simulink model "UPS_3level_Ttype_Inverter_simplified_ctrl"  (R2012b)
settings: Solver=ode4  StartTime=0.0  StopTime=Tfinal  FixedStep=Ts  MaxStep=1e-5  RelTol=1e-3
values from neighbouring files (symbols this model uses):
  Ts = 1/(1*1e6)    (= 1e-06)    [Run.m]
  Vd = 720    [Run.m]
  VSI = rmfield(VSI, {'IF1', 'IF2', 'FLUXlin1', 'FLUXlin2',      'FLUXnonlin1', 'FLUXnonlin2', 'Lfnonlin'})    [Run.m]
undefined symbols (not defined in the file or in its folder): ADC, CTRL, DiscIntNeverNeededParam, PR, S, UPS
libraries: powerlib x113, simulink_extras x11, powerlib_extras x11, simulink x3
(part 1 of 3)
CloseFcn:
  | rtwprivate ssgencode ModelCloseRequest AC_DC_3f_400k_PW
settings Model: BufferReuse=off  Creator=Adam  LastModifiedBy=chstalm
settings DataIOCC: SignalLoggingSaveFormat=ModelDataLogs  InspectSignalLogs=on
settings OptimizationCC: BlockReduction=off  InlineParams=on  BufferReuse=off  InitFltsAndDblsToZero=on
settings DebuggingCC: SaveWithParameterizedLinksMsg=none  CheckSSInitialOutputMsg=off  SignalResolutionControl=TryResolveAllWithWarning  FcnCallInpInsideContextMsg=UseLocalSettings  UnconnectedInputMsg=none  UnconnectedOutputMsg=none  UnconnectedLineMsg=none  StrictBusMsg=Warning
settings GRTTargetCC: TargetFcnLib=ansi_tfl_tmw.mat  CombineOutputUpdateFcns=off  GRTInterface=on

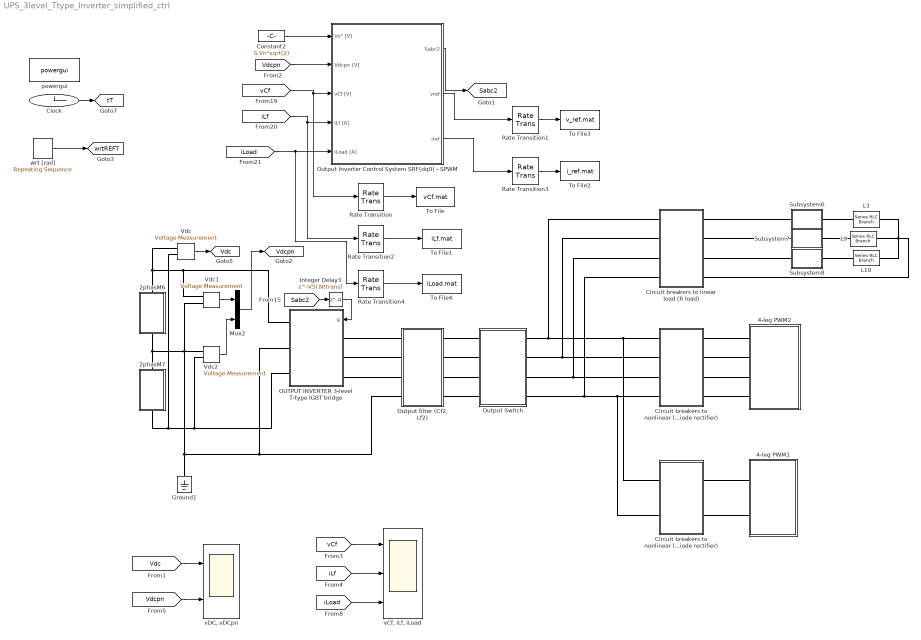
== system UPS_3level_Ttype_Inverter_simplified_ctrl ==
  2phasM6 : Subsystem
  2phasM7 : Subsystem
  4-leg PWM1 : Subsystem
  4-leg PWM2 : Subsystem
  Circuit breakers to linear load (R load) : Subsystem
  Circuit breakers to nonlinear load (1-phase diode rectifier) : Subsystem
  Circuit breakers to nonlinear load (3-phase diode rectifier) : Subsystem
  Clock : Clock
  Constant2 : Constant  Value=S.Vn*sqrt(2)  SampleTime=Ts
  Ground1 : powerlib/Elements/Ground  LConnTagsString=a
  Integer Delay3 : Delay  DelayLength=VSI.Nttransf  InitialCondition=0  InputProcessing=Inherited
  L10 : powerlib/Elements/Series RLC Branch  LConnTagsString=__new0  RConnTagsString=__new0  BranchType=RL  Resistance=VSI.Rc  Inductance=VSI.Lc  SetiL0=off  InitialCurrent=0  Capacitance=1.0  Setx0=off  InitialVoltage=0  Measurements=None
  L3 : powerlib/Elements/Series RLC Branch  LConnTagsString=__new0  RConnTagsString=__new0  BranchType=RL  Resistance=VSI.Ra  Inductance=VSI.La  SetiL0=off  InitialCurrent=0  Capacitance=1.0  Setx0=off  InitialVoltage=0  Measurements=None
  L9 : powerlib/Elements/Series RLC Branch  LConnTagsString=__new0  RConnTagsString=__new0  BranchType=RL  Resistance=VSI.Rb  Inductance=VSI.Lb  SetiL0=off  InitialCurrent=0  Capacitance=1.0  Setx0=off  InitialVoltage=0  Measurements=None
  Mux2 : Mux  Inputs=2
  OUTPUT INVERTER 3-level T-type IGBT bridge : Subsystem
  Output Switch : Subsystem
  "Output Inverter Control System SRF(dq0) - SPWM " : Subsystem
  "Output filter (Cf2, Lf2)" : Subsystem
  Rate Transition{,1..4} (5 alike) : RateTransition  OutPortSampleTime=1e-5
  Subsystem6 : Subsystem
  Subsystem7 : Subsystem
  Subsystem8 : Subsystem
  To File : ToFile  Filename=vCf.mat  MatrixName=vCf  SaveFormat=Timeseries
  To File1 : ToFile  Filename=iLf.mat  MatrixName=iLf  SaveFormat=Timeseries
  To File2 : ToFile  Filename=i_ref.mat  MatrixName=i_ref  SaveFormat=Timeseries
  To File3 : ToFile  Filename=v_ref.mat  MatrixName=v_ref  SaveFormat=Timeseries
  To File4 : ToFile  Filename=iLoad.mat  MatrixName=iLoad  SaveFormat=Timeseries
  Vdc : powerlib/Measurements/Voltage Measurement  PhasorSimulation=off  OutputType=Complex  PSBequivalent=0
  Vdc1 : powerlib/Measurements/Voltage Measurement  PhasorSimulation=off  OutputType=Complex  PSBequivalent=0
  Vdc2 : powerlib/Measurements/Voltage Measurement  PhasorSimulation=off  OutputType=Complex  PSBequivalent=0
  powergui : powerlib/powergui  SimulationMode=Discrete  SolverType=Tustin  SampleTime=Ts  frequency=60  SPID=off  DisableSnubberDevices=off  DisableRonSwitches=off  DisableVfSwitches=off  SwTol=0  Interpol=off  DisplayEquations=off  FunctionMessages=off  frequencyindice=0  Pbase=100e6  ErrMax=1e-4  Iterations=50  UnitsV=kV  UnitsW=MW  echomessages=off  HookPort=off  EnableUseOfTLC=off  x0status=blocks  RestoreLinks=warning  ResistiveCurrentMeasurement=off  Frange=[0:2:500]  Ylog=off  Xlog=on  ShowGrid=off  save=off  variable=ZData  ZoomFFT=on  StartTime=0.0  cycles=1  DisplayStyle=1  fundamental=60  FreqAxis=off  MaxFrequency=1000  frequencyindicesteady=1  RmsSteady=1  display=off  Ts=0  methode=off
  "vCf, iLf, iLoad" : Scope  NumInputPorts=3
      settings: TimeRange=0.7000000000000001  YMin=-500~-400~-400  YMax=500~400~400  SaveName=VSIout  DataFormat=Structure  Decimation=10  SampleInput=on
  "vDC, vDCpn" : Scope  NumInputPorts=2
      settings: TimeRange=0.1738072054527751  YMin=0~0  YMax=750~375  SaveName=Rectifier_in1  DataFormat=Structure  Decimation=10  SampleInput=on
  wrt [rad] : simulink/Sources/Repeating Sequence  rep_seq_t="[0    1/S.fn]"  rep_seq_y="[0    2*pi]"
  tag scope: Sabc2=global, Vdc=global, Vdcpn=global, tT=global, wrtREFT=global
  wires:
  Clock/1 -> [tT]
  [Sabc2] -> Integer Delay3/1
  [Vdcpn] -> "Output Inverter Control System SRF(dq0) - SPWM "/2(Vdcpn [V])
  [vCf] -> Rate Transition/1, "Output Inverter Control System SRF(dq0) - SPWM "/3(vCf [V])
  [iLf] -> Rate Transition2/1, "Output Inverter Control System SRF(dq0) - SPWM "/4(iLf [A])
  "Output Inverter Control System SRF(dq0) - SPWM "/1(Sabc2) -> [Sabc2]
  [iLoad] -> Rate Transition4/1, "Output Inverter Control System SRF(dq0) - SPWM "/5(iLoad [A])
  Integer Delay3/1 -> OUTPUT INVERTER 3-level T-type IGBT bridge/1(g)
  Vdc/1 -> [Vdc]
  [vCf] -> "vCf, iLf, iLoad"/1
  [iLoad] -> "vCf, iLf, iLoad"/3
  [iLf] -> "vCf, iLf, iLoad"/2
  Vdc1/1 -> Mux2/1
  Vdc2/1 -> Mux2/2
  Mux2/1 -> [Vdcpn]
  [Vdcpn] -> "vDC, vDCpn"/2
  [Vdc] -> "vDC, vDCpn"/1
  wrt [rad]/1 -> [wrtREFT]
  Rate Transition/1 -> To File/1
  Rate Transition1/1 -> To File3/1
  "Output Inverter Control System SRF(dq0) - SPWM "/2(vref) -> Rate Transition1/1
  Constant2/1 -> "Output Inverter Control System SRF(dq0) - SPWM "/1(Vs* [V])
  Rate Transition2/1 -> To File1/1
  Rate Transition3/1 -> To File2/1
  "Output Inverter Control System SRF(dq0) - SPWM "/3(iref) -> Rate Transition3/1
  Rate Transition4/1 -> To File4/1
  connections:
  Output Switch/LConn1 -- "Output filter (Cf2, Lf2)"/RConn1
  Output Switch/LConn2 -- "Output filter (Cf2, Lf2)"/RConn2
  Output Switch/LConn4 -- "Output filter (Cf2, Lf2)"/RConn4
  Output Switch/LConn3 -- "Output filter (Cf2, Lf2)"/RConn3
  Vdc2/LConn2 -- OUTPUT INVERTER 3-level T-type IGBT bridge/RConn3 -- 2phasM7/RConn1 -- Vdc/LConn2
  Vdc1/LConn1 -- OUTPUT INVERTER 3-level T-type IGBT bridge/RConn1 -- 2phasM6/LConn1 -- Vdc/LConn1
  OUTPUT INVERTER 3-level T-type IGBT bridge/LConn1 -- "Output filter (Cf2, Lf2)"/LConn1
  OUTPUT INVERTER 3-level T-type IGBT bridge/LConn2 -- "Output filter (Cf2, Lf2)"/LConn2
  OUTPUT INVERTER 3-level T-type IGBT bridge/LConn3 -- "Output filter (Cf2, Lf2)"/LConn3
  OUTPUT INVERTER 3-level T-type IGBT bridge/RConn2 -- "Output filter (Cf2, Lf2)"/LConn4 -- Ground1/LConn1 -- Vdc2/LConn1 -- Vdc1/LConn2 -- 2phasM7/LConn1 -- 2phasM6/RConn1
  Subsystem6/RConn1 -- L3/LConn1
  Subsystem8/RConn1 -- L10/LConn1
  Subsystem7/RConn1 -- L9/LConn1
  Circuit breakers to linear load (R load)/RConn1 -- Subsystem6/LConn1
  Circuit breakers to linear load (R load)/RConn2 -- Subsystem7/LConn1
  Circuit breakers to linear load (R load)/RConn3 -- Subsystem8/LConn1
  L10/RConn1 -- L3/RConn1 -- L9/RConn1 -- Circuit breakers to linear load (R load)/RConn4
  Circuit breakers to nonlinear load (3-phase diode rectifier)/RConn1 -- 4-leg PWM2/LConn1
  Circuit breakers to nonlinear load (3-phase diode rectifier)/RConn2 -- 4-leg PWM2/LConn2
  Circuit breakers to nonlinear load (3-phase diode rectifier)/RConn3 -- 4-leg PWM2/LConn3
  Circuit breakers to nonlinear load (3-phase diode rectifier)/RConn4 -- 4-leg PWM2/LConn4
  4-leg PWM1/LConn1 -- Circuit breakers to nonlinear load (1-phase diode rectifier)/RConn1
  4-leg PWM1/LConn2 -- Circuit breakers to nonlinear load (1-phase diode rectifier)/RConn2
  Output Switch/RConn1 -- Circuit breakers to nonlinear load (1-phase diode rectifier)/LConn1 -- Circuit breakers to nonlinear load (3-phase diode rectifier)/LConn1 -- Circuit breakers to linear load (R load)/LConn1
  Output Switch/RConn2 -- Circuit breakers to nonlinear load (3-phase diode rectifier)/LConn2 -- Circuit breakers to linear load (R load)/LConn2
  Output Switch/RConn3 -- Circuit breakers to nonlinear load (3-phase diode rectifier)/LConn3 -- Circuit breakers to linear load (R load)/LConn3
  Output Switch/RConn4 -- Circuit breakers to nonlinear load (1-phase diode rectifier)/LConn2 -- Circuit breakers to nonlinear load (3-phase diode rectifier)/LConn4 -- Circuit breakers to linear load (R load)/LConn4

== system UPS_3level_Ttype_Inverter_simplified_ctrl/2phasM6 ==
  DC Voltage Source : powerlib/Electrical Sources/DC Voltage Source  Amplitude=Vd/2  Measurements=None
  Vd1 : powerlib/Measurements/Voltage Measurement  PhasorSimulation=off  OutputType=Complex  PSBequivalent=0
  DC+ : PMIOPort  Port=1  Side=Left
  n : PMIOPort  Port=2  Side=Right
  tag scope: Vd1T=global
  wires:
  Vd1/1 -> [Vd1T]
  connections:
  DC+/RConn1 -- DC Voltage Source/RConn1 -- Vd1/LConn1
  n/RConn1 -- DC Voltage Source/LConn1 -- Vd1/LConn2

== system UPS_3level_Ttype_Inverter_simplified_ctrl/2phasM7 ==
  DC Voltage Source : powerlib/Electrical Sources/DC Voltage Source  Amplitude=Vd/2  Measurements=None
  Vd2 : powerlib/Measurements/Voltage Measurement  PhasorSimulation=off  OutputType=Complex  PSBequivalent=0
  n : PMIOPort  Port=1  Side=Left
  DC- : PMIOPort  Port=2  Side=Right
  tag scope: Vd2T=global
  wires:
  Vd2/1 -> [Vd2T]
  connections:
  n/RConn1 -- DC Voltage Source/RConn1 -- Vd2/LConn1
  DC-/RConn1 -- DC Voltage Source/LConn1 -- Vd2/LConn2

== system UPS_3level_Ttype_Inverter_simplified_ctrl/4-leg PWM1 ==
  D{1..2,7..8} (4 alike) : powerlib/Power Electronics/Diode  Ron=1e-3  Lon=0  Vf=0.8  IC=0  UseSnubber=off  Rs=1e6  Cs=inf  Measurements=off
  L1 : powerlib/Elements/Series RLC Branch  LConnTagsString=__new0  RConnTagsString=__new0  BranchType=R  Resistance=VSI.DR_Rs  Inductance=VSI.La  SetiL0=off  InitialCurrent=0  Capacitance=1.0  Setx0=off  InitialVoltage=0  Measurements=None
  L7 : powerlib/Elements/Series RLC Branch  LConnTagsString=__new0  RConnTagsString=__new0  BranchType=R  Resistance=VSI.DR_Rload  Inductance=VSI.La  SetiL0=off  InitialCurrent=0  Capacitance=1.0  Setx0=off  InitialVoltage=0  Measurements=None
  Series RLC Branch1 : powerlib/Elements/Series RLC Branch  LConnTagsString=__new0  RConnTagsString=__new0  BranchType=C  Resistance=1  Inductance=1e-3  SetiL0=off  InitialCurrent=0  Capacitance=VSI.DR_C  Setx0=on  InitialVoltage=VSI.DR_Vc0  Measurements=None
  Subsystem3 : Subsystem
  A : PMIOPort  Tag=PMCPort  Port=1  Side=Left
  N : PMIOPort  Tag=PMCPort  Port=2  Side=Left
  connections:
  D1/RConn1 -- Series RLC Branch1/LConn1 -- L7/LConn1 -- D7/RConn1
  D2/RConn1 -- L1/LConn1 -- D1/LConn1
  D8/LConn1 -- Series RLC Branch1/RConn1 -- L7/RConn1 -- D2/LConn1
  Subsystem3/LConn1 -- A/RConn1
  Subsystem3/RConn1 -- L1/RConn1
  D8/RConn1 -- N/RConn1 -- D7/LConn1

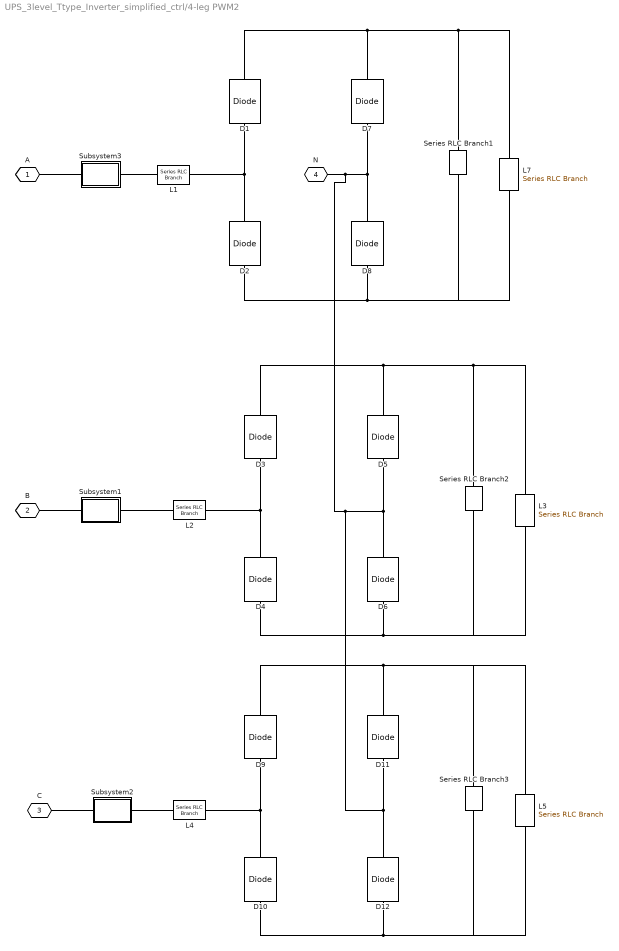
== system UPS_3level_Ttype_Inverter_simplified_ctrl/4-leg PWM2 ==
  D{1..12} (12 alike) : powerlib/Power Electronics/Diode  Ron=1e-3  Lon=0  Vf=0.8  IC=0  UseSnubber=off  Rs=1e6  Cs=inf  Measurements=off
  L1 : powerlib/Elements/Series RLC Branch  LConnTagsString=__new0  RConnTagsString=__new0  BranchType=R  Resistance=VSI.DR_Rs  Inductance=VSI.La  SetiL0=off  InitialCurrent=0  Capacitance=1.0  Setx0=off  InitialVoltage=0  Measurements=None
  L2 : powerlib/Elements/Series RLC Branch  LConnTagsString=__new0  RConnTagsString=__new0  BranchType=R  Resistance=VSI.DR_Rs  Inductance=VSI.La  SetiL0=off  InitialCurrent=0  Capacitance=1.0  Setx0=off  InitialVoltage=0  Measurements=None
  L3 : powerlib/Elements/Series RLC Branch  LConnTagsString=__new0  RConnTagsString=__new0  BranchType=R  Resistance=VSI.DR_Rload  Inductance=VSI.La  SetiL0=off  InitialCurrent=0  Capacitance=1.0  Setx0=off  InitialVoltage=0  Measurements=None
  L4 : powerlib/Elements/Series RLC Branch  LConnTagsString=__new0  RConnTagsString=__new0  BranchType=R  Resistance=VSI.DR_Rs  Inductance=VSI.La  SetiL0=off  InitialCurrent=0  Capacitance=1.0  Setx0=off  InitialVoltage=0  Measurements=None
  L5 : powerlib/Elements/Series RLC Branch  LConnTagsString=__new0  RConnTagsString=__new0  BranchType=R  Resistance=VSI.DR_Rload  Inductance=VSI.La  SetiL0=off  InitialCurrent=0  Capacitance=1.0  Setx0=off  InitialVoltage=0  Measurements=None
  L7 : powerlib/Elements/Series RLC Branch  LConnTagsString=__new0  RConnTagsString=__new0  BranchType=R  Resistance=VSI.DR_Rload  Inductance=VSI.La  SetiL0=off  InitialCurrent=0  Capacitance=1.0  Setx0=off  InitialVoltage=0  Measurements=None
  Series RLC Branch1 : powerlib/Elements/Series RLC Branch  LConnTagsString=__new0  RConnTagsString=__new0  BranchType=C  Resistance=1  Inductance=1e-3  SetiL0=off  InitialCurrent=0  Capacitance=VSI.DR_C  Setx0=on  InitialVoltage=VSI.DR_Vc0  Measurements=None
  Series RLC Branch2 : powerlib/Elements/Series RLC Branch  LConnTagsString=__new0  RConnTagsString=__new0  BranchType=C  Resistance=1  Inductance=1e-3  SetiL0=off  InitialCurrent=0  Capacitance=VSI.DR_C  Setx0=on  InitialVoltage=VSI.DR_Vc0  Measurements=None
  Series RLC Branch3 : powerlib/Elements/Series RLC Branch  LConnTagsString=__new0  RConnTagsString=__new0  BranchType=C  Resistance=1  Inductance=1e-3  SetiL0=off  InitialCurrent=0  Capacitance=VSI.DR_C  Setx0=on  InitialVoltage=VSI.DR_Vc0  Measurements=None
  Subsystem1 : Subsystem
  Subsystem2 : Subsystem
  Subsystem3 : Subsystem
  A : PMIOPort  Tag=PMCPort  Port=1  Side=Left
  B : PMIOPort  Tag=PMCPort  Port=2  Side=Left
  C : PMIOPort  Tag=PMCPort  Port=3  Side=Left
  N : PMIOPort  Tag=PMCPort  Port=4  Side=Left
  connections:
  D1/RConn1 -- L7/LConn1 -- Series RLC Branch1/LConn1 -- D7/RConn1
  D2/RConn1 -- L1/LConn1 -- D1/LConn1
  D8/LConn1 -- L7/RConn1 -- Series RLC Branch1/RConn1 -- D2/LConn1
  D4/RConn1 -- L2/LConn1 -- D3/LConn1
  D6/LConn1 -- L3/RConn1 -- Series RLC Branch2/RConn1 -- D4/LConn1
  D9/RConn1 -- Series RLC Branch3/LConn1 -- L5/LConn1 -- D11/RConn1
  D10/RConn1 -- L4/LConn1 -- D9/LConn1
  D12/LConn1 -- L5/RConn1 -- Series RLC Branch3/RConn1 -- D10/LConn1
  D3/RConn1 -- L3/LConn1 -- Series RLC Branch2/LConn1 -- D5/RConn1
  Subsystem2/LConn1 -- C/RConn1
  Subsystem1/LConn1 -- B/RConn1
  Subsystem3/LConn1 -- A/RConn1
  Subsystem3/RConn1 -- L1/RConn1
  D12/RConn1 -- D11/LConn1 -- D6/RConn1 -- D5/LConn1 -- D8/RConn1 -- D7/LConn1 -- N/RConn1
  L2/RConn1 -- Subsystem1/RConn1
  L4/RConn1 -- Subsystem2/RConn1

== system UPS_3level_Ttype_Inverter_simplified_ctrl/Circuit breakers to linear load (R load) ==
  Branch_C : MultiPortSwitch  Inputs=4  SaturateOnIntegerOverflow=on  InputSameDT=on
  Constant1 : Constant  Value=[1 0 0 1]
  Constant2 : Constant  Value=UPS.LoadR123 + 1
  Constant3 : Constant  Value=[1 1 0 1]
  Constant4 : Constant  Value=[1 1 1 1]
  Constant5 : Constant  Value=[0 0 0 0]
  Data Type Conversion{1..4} (4 alike) : DataTypeConversion  OutDataTypeStr=boolean  SaturateOnIntegerOverflow=on  RndMeth=Zero
  Demux : Demux
  Ideal Switch{,1..3} (4 alike) : powerlib/Power Electronics/Ideal Switch  Ron=0.001  Lon=0  IC=0  Rs=1e6  Cs=inf  Measurements=off
  A2 : PMIOPort  Port=1  Side=Left
  B2 : PMIOPort  Port=2  Side=Left
  C2 : PMIOPort  Port=3  Side=Left
  N2 : PMIOPort  Port=4  Side=Left
  a2 : PMIOPort  Port=5  Side=Right
  b2 : PMIOPort  Port=6  Side=Right
  c2 : PMIOPort  Port=7  Side=Right
  n2 : PMIOPort  Port=8  Side=Right
  wires:
  Constant4/1 -> Branch_C/5
  Constant3/1 -> Branch_C/4
  Constant1/1 -> Branch_C/3
  Constant5/1 -> Branch_C/2
  Constant2/1 -> Branch_C/1
  Branch_C/1 -> Demux/1
  Data Type Conversion2/1 -> Ideal Switch3/1
  Data Type Conversion1/1 -> Ideal Switch2/1
  Data Type Conversion3/1 -> Ideal Switch1/1
  Data Type Conversion4/1 -> Ideal Switch/1
  Demux/1 -> Data Type Conversion2/1
  Demux/2 -> Data Type Conversion1/1
  Demux/3 -> Data Type Conversion3/1
  Demux/4 -> Data Type Conversion4/1
  connections:
  Ideal Switch/LConn1 -- N2/RConn1
  n2/RConn1 -- Ideal Switch/RConn1
  Ideal Switch1/LConn1 -- C2/RConn1
  Ideal Switch1/RConn1 -- c2/RConn1
  Ideal Switch2/LConn1 -- B2/RConn1
  Ideal Switch2/RConn1 -- b2/RConn1
  Ideal Switch3/LConn1 -- A2/RConn1
  Ideal Switch3/RConn1 -- a2/RConn1

== system UPS_3level_Ttype_Inverter_simplified_ctrl/Circuit breakers to nonlinear load (1-phase diode rectifier) ==
  Constant2 : Constant  Value=UPS.LoadD1
  Data Type Conversion2 : DataTypeConversion  OutDataTypeStr=boolean  SaturateOnIntegerOverflow=on  RndMeth=Zero
  Ideal Switch2 : powerlib/Power Electronics/Ideal Switch  Ron=0.001  Lon=0  IC=0  Rs=1e6  Cs=inf  Measurements=off
  Ideal Switch3 : powerlib/Power Electronics/Ideal Switch  Ron=0.001  Lon=0  IC=0  Rs=1e6  Cs=inf  Measurements=off
  A2 : PMIOPort  Port=1  Side=Left
  N2 : PMIOPort  Port=2  Side=Left
  a2 : PMIOPort  Port=3  Side=Right
  n2 : PMIOPort  Port=4  Side=Right
  wires:
  Constant2/1 -> Data Type Conversion2/1
  Data Type Conversion2/1 -> Ideal Switch3/1, Ideal Switch2/1
  connections:
  Ideal Switch2/LConn1 -- N2/RConn1
  Ideal Switch2/RConn1 -- n2/RConn1
  Ideal Switch3/LConn1 -- A2/RConn1
  Ideal Switch3/RConn1 -- a2/RConn1

== system UPS_3level_Ttype_Inverter_simplified_ctrl/Circuit breakers to nonlinear load (3-phase diode rectifier) ==
  Constant2 : Constant  Value=UPS.LoadD3
  Data Type Conversion2 : DataTypeConversion  OutDataTypeStr=boolean  SaturateOnIntegerOverflow=on  RndMeth=Zero
  Ideal Switch{,1..3} (4 alike) : powerlib/Power Electronics/Ideal Switch  Ron=0.001  Lon=0  IC=0  Rs=1e6  Cs=inf  Measurements=off
  A2 : PMIOPort  Port=1  Side=Left
  B2 : PMIOPort  Port=2  Side=Left
  C2 : PMIOPort  Port=3  Side=Left
  N2 : PMIOPort  Port=4  Side=Left
  a2 : PMIOPort  Port=5  Side=Right
  b2 : PMIOPort  Port=6  Side=Right
  c2 : PMIOPort  Port=7  Side=Right
  n2 : PMIOPort  Port=8  Side=Right
  wires:
  Constant2/1 -> Data Type Conversion2/1
  Data Type Conversion2/1 -> Ideal Switch3/1, Ideal Switch2/1, Ideal Switch1/1, Ideal Switch/1
  connections:
  Ideal Switch/LConn1 -- N2/RConn1
  n2/RConn1 -- Ideal Switch/RConn1
  Ideal Switch1/LConn1 -- C2/RConn1
  Ideal Switch1/RConn1 -- c2/RConn1
  Ideal Switch2/LConn1 -- B2/RConn1
  Ideal Switch2/RConn1 -- b2/RConn1
  Ideal Switch3/LConn1 -- A2/RConn1
  Ideal Switch3/RConn1 -- a2/RConn1

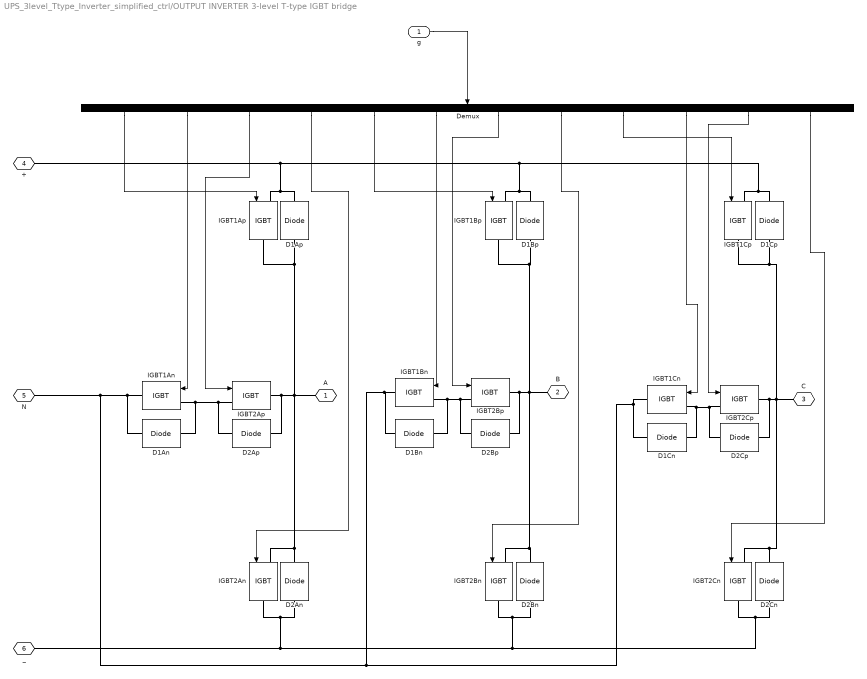
== system UPS_3level_Ttype_Inverter_simplified_ctrl/OUTPUT INVERTER 3-level T-type IGBT bridge ==
  g : Inport
  D1An : powerlib/Power Electronics/Diode  Ron=1e-3  Lon=0  Vf=0.8  IC=0  UseSnubber=off  Rs=inf  Cs=0  Measurements=off
  D1Ap : powerlib/Power Electronics/Diode  Ron=1e-3  Lon=0  Vf=0.8  IC=0  UseSnubber=off  Rs=inf  Cs=0  Measurements=off
  D1Bn : powerlib/Power Electronics/Diode  Ron=1e-3  Lon=0  Vf=0.8  IC=0  UseSnubber=off  Rs=inf  Cs=0  Measurements=off
  D1Bp : powerlib/Power Electronics/Diode  Ron=1e-3  Lon=0  Vf=0.8  IC=0  UseSnubber=off  Rs=inf  Cs=0  Measurements=off
  D1Cn : powerlib/Power Electronics/Diode  Ron=1e-3  Lon=0  Vf=0.8  IC=0  UseSnubber=off  Rs=inf  Cs=0  Measurements=off
  D1Cp : powerlib/Power Electronics/Diode  Ron=1e-3  Lon=0  Vf=0.8  IC=0  UseSnubber=off  Rs=inf  Cs=0  Measurements=off
  D2An : powerlib/Power Electronics/Diode  Ron=1e-3  Lon=0  Vf=0.8  IC=0  UseSnubber=off  Rs=inf  Cs=0  Measurements=off
  D2Ap : powerlib/Power Electronics/Diode  Ron=1e-3  Lon=0  Vf=0.8  IC=0  UseSnubber=off  Rs=inf  Cs=0  Measurements=off
  D2Bn : powerlib/Power Electronics/Diode  Ron=1e-3  Lon=0  Vf=0.8  IC=0  UseSnubber=off  Rs=inf  Cs=0  Measurements=off
  D2Bp : powerlib/Power Electronics/Diode  Ron=1e-3  Lon=0  Vf=0.8  IC=0  UseSnubber=off  Rs=inf  Cs=0  Measurements=off
  D2Cn : powerlib/Power Electronics/Diode  Ron=1e-3  Lon=0  Vf=0.8  IC=0  UseSnubber=off  Rs=inf  Cs=0  Measurements=off
  D2Cp : powerlib/Power Electronics/Diode  Ron=1e-3  Lon=0  Vf=0.8  IC=0  UseSnubber=off  Rs=inf  Cs=0  Measurements=off
  Demux : Demux  Outputs=12
  IGBT1An : powerlib/Power Electronics/IGBT  Ron=1e-3  Lon=0  Vf=1  Tf=0  Tt=0  IC=0  Rs=1e5  Cs=inf  Measurements=off
  IGBT1Ap : powerlib/Power Electronics/IGBT  Ron=1e-3  Lon=0  Vf=1  Tf=0  Tt=0  IC=0  Rs=1e5  Cs=inf  Measurements=off
  IGBT1Bn : powerlib/Power Electronics/IGBT  Ron=1e-3  Lon=0  Vf=1  Tf=0  Tt=0  IC=0  Rs=1e5  Cs=inf  Measurements=off
  IGBT1Bp : powerlib/Power Electronics/IGBT  Ron=1e-3  Lon=0  Vf=1  Tf=0  Tt=0  IC=0  Rs=1e5  Cs=inf  Measurements=off
  IGBT1Cn : powerlib/Power Electronics/IGBT  Ron=1e-3  Lon=0  Vf=1  Tf=0  Tt=0  IC=0  Rs=1e5  Cs=inf  Measurements=off
  IGBT1Cp : powerlib/Power Electronics/IGBT  Ron=1e-3  Lon=0  Vf=1  Tf=0  Tt=0  IC=0  Rs=1e5  Cs=inf  Measurements=off
  IGBT2An : powerlib/Power Electronics/IGBT  Ron=1e-3  Lon=0  Vf=1  Tf=0  Tt=0  IC=0  Rs=1e5  Cs=inf  Measurements=off
  IGBT2Ap : powerlib/Power Electronics/IGBT  Ron=1e-3  Lon=0  Vf=1  Tf=0  Tt=0  IC=0  Rs=1e5  Cs=inf  Measurements=off
  IGBT2Bn : powerlib/Power Electronics/IGBT  Ron=1e-3  Lon=0  Vf=1  Tf=0  Tt=0  IC=0  Rs=1e5  Cs=inf  Measurements=off
  IGBT2Bp : powerlib/Power Electronics/IGBT  Ron=1e-3  Lon=0  Vf=1  Tf=0  Tt=0  IC=0  Rs=1e5  Cs=inf  Measurements=off
  IGBT2Cn : powerlib/Power Electronics/IGBT  Ron=1e-3  Lon=0  Vf=1  Tf=0  Tt=0  IC=0  Rs=1e5  Cs=inf  Measurements=off
  IGBT2Cp : powerlib/Power Electronics/IGBT  Ron=1e-3  Lon=0  Vf=1  Tf=0  Tt=0  IC=0  Rs=1e5  Cs=inf  Measurements=off
  A : PMIOPort  Tag=PMCPort  Port=1  Side=Left
  B : PMIOPort  Tag=PMCPort  Port=2  Side=Left
  C : PMIOPort  Tag=PMCPort  Port=3  Side=Left
  + : PMIOPort  Tag=PMCPort  Port=4  Side=Right
  N : PMIOPort  Tag=PMCPort  Port=5  Side=Right
  _ : PMIOPort  Tag=PMCPort  Port=6  Side=Right
  wires:
  g/1 -> Demux/1
  Demux/1 -> IGBT1Ap/1
  Demux/2 -> IGBT1An/1
  Demux/3 -> IGBT2Ap/1
  Demux/4 -> IGBT2An/1
  Demux/5 -> IGBT1Bp/1
  Demux/6 -> IGBT1Bn/1
  Demux/7 -> IGBT2Bp/1
  Demux/8 -> IGBT2Bn/1
  Demux/9 -> IGBT1Cp/1
  Demux/10 -> IGBT1Cn/1
  Demux/11 -> IGBT2Cp/1
  Demux/12 -> IGBT2Cn/1
  connections:
  IGBT1Cp/LConn1 -- D1Cp/RConn1 -- IGBT1Ap/LConn1 -- D1Ap/RConn1 -- +/RConn1 -- D1Bp/RConn1 -- IGBT1Bp/LConn1
  IGBT2Ap/LConn1 -- D2Ap/RConn1 -- IGBT1An/LConn1 -- D1An/RConn1
  IGBT1Cp/RConn1 -- D1Cp/LConn1 -- D2Cp/LConn1 -- IGBT2Cp/RConn1 -- C/RConn1 -- IGBT2Cn/LConn1 -- D2Cn/RConn1
  IGBT2Cn/RConn1 -- D2Cn/LConn1 -- _/RConn1 -- IGBT2An/RConn1 -- D2An/LConn1 -- IGBT2Bn/RConn1 -- D2Bn/LConn1
  IGBT1Ap/RConn1 -- D1Ap/LConn1 -- IGBT2An/LConn1 -- D2An/RConn1 -- A/RConn1 -- IGBT2Ap/RConn1 -- D2Ap/LConn1
  D2Bp/RConn1 -- IGBT2Bp/LConn1 -- IGBT1Bn/LConn1 -- D1Bn/RConn1
  D2Bn/RConn1 -- IGBT2Bn/LConn1 -- D1Bp/LConn1 -- IGBT1Bp/RConn1 -- D2Bp/LConn1 -- IGBT2Bp/RConn1 -- B/RConn1
  D2Cp/RConn1 -- IGBT2Cp/LConn1 -- D1Cn/RConn1 -- IGBT1Cn/LConn1
  IGBT1Cn/RConn1 -- IGBT1An/RConn1 -- D1An/LConn1 -- N/RConn1 -- IGBT1Bn/RConn1 -- D1Bn/LConn1 -- D1Cn/LConn1

== system UPS_3level_Ttype_Inverter_simplified_ctrl/Output Switch ==
  2 [s]1 : Constant  Value=VSI.ton
  2 [s]5 : Constant  Value=VSI.tk
  Logical Operator : Logic  AllPortsSameDT=off  OutDataTypeStr=boolean
  Relational Operator1 : RelationalOperator  OutDataTypeStr=boolean
  Relational Operator3 : RelationalOperator  Operator=<=  OutDataTypeStr=boolean
  Subsystem4 : Subsystem
  Subsystem5 : Subsystem
  Subsystem7 : Subsystem
  A2 : PMIOPort  Port=1  Side=Left
  B2 : PMIOPort  Port=2  Side=Left
  a2 : PMIOPort  Port=3  Side=Right
  b2 : PMIOPort  Port=4  Side=Right
  C2 : PMIOPort  Port=5  Side=Left
  c2 : PMIOPort  Port=6  Side=Right
  N2 : PMIOPort  Port=7  Side=Left
  n2 : PMIOPort  Port=8  Side=Right
  wires:
  2 [s]1/1 -> Relational Operator1/2
  Relational Operator1/1 -> Logical Operator/1
  Relational Operator3/1 -> Logical Operator/2
  2 [s]5/1 -> Relational Operator3/2
  [tT] -> Relational Operator1/1, Relational Operator3/1
  Logical Operator/1 -> Subsystem5/1(on/off), Subsystem4/1(on/off), Subsystem7/1(on/off)
  connections:
  Subsystem4/RConn1 -- b2/RConn1
  N2/RConn1 -- n2/RConn1
  Subsystem7/RConn1 -- a2/RConn1
  Subsystem5/RConn1 -- c2/RConn1
  C2/RConn1 -- Subsystem5/LConn1
  B2/RConn1 -- Subsystem4/LConn1
  A2/RConn1 -- Subsystem7/LConn1

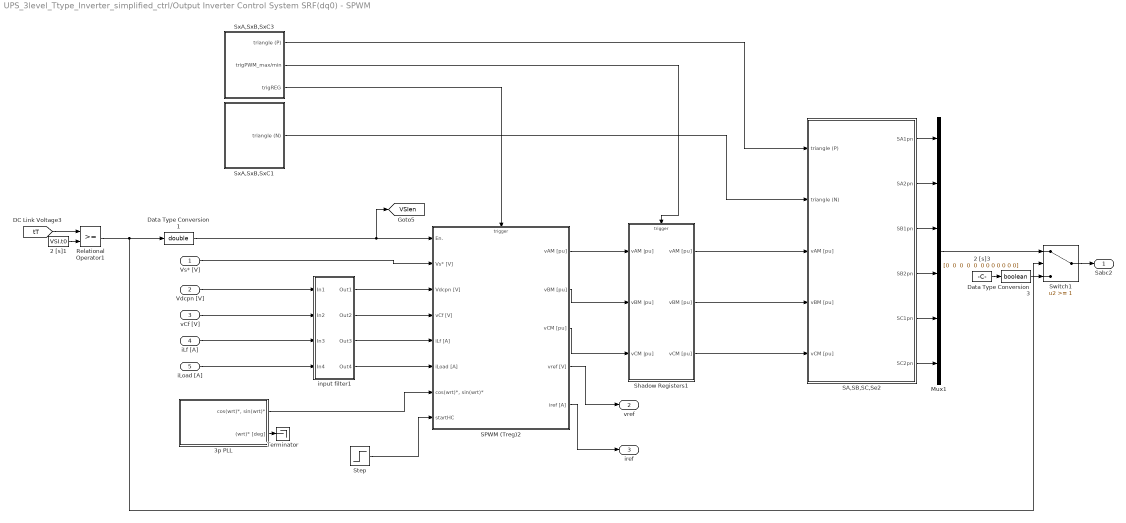
== system UPS_3level_Ttype_Inverter_simplified_ctrl/Output Inverter Control System SRF(dq0) - SPWM  ==
  Vs* [V] : Inport
  Vdcpn [V] : Inport  Port=2
  vCf [V] : Inport  Port=3
  iLf [A] : Inport  Port=4
  iLoad [A] : Inport  Port=5
  2 [s]1 : Constant  Value=VSI.t0
  2 [s]3 : Constant  Value="[0  0  0  0  0  0 0 0 0 0 0 0]"
  3p PLL : Subsystem
  Data Type Conversion1 : DataTypeConversion  OutDataTypeStr=double  SaturateOnIntegerOverflow=on  RndMeth=Zero
  Data Type Conversion3 : DataTypeConversion  OutDataTypeStr=boolean  SaturateOnIntegerOverflow=on  RndMeth=Zero
  Mux1 : Mux  Inputs=6
  Relational Operator1 : RelationalOperator  OutDataTypeStr=boolean
  SA,SB,SC,Se2 : Subsystem
  SPWM (Treg)2 : Subsystem
  Shadow Registers1 : Subsystem
  Step : Step  Time=0.1  SampleTime=0
  Switch1 : Switch  Threshold=1
  SxA,SxB,SxC1 : Subsystem
  SxA,SxB,SxC3 : Subsystem
  Terminator : Terminator
  input filter1 : Subsystem
  Sabc2 : Outport
  vref : Outport  Port=2
  iref : Outport  Port=3
  tag scope: VSIen=global
  wires:
  2 [s]3/1 -> Data Type Conversion3/1
  Data Type Conversion3/1 -> Switch1/3
  [tT] -> Relational Operator1/1
  2 [s]1/1 -> Relational Operator1/2
  Relational Operator1/1 -> Data Type Conversion1/1, Switch1/2
  Mux1/1 -> Switch1/1
  Switch1/1 -> Sabc2/1
  3p PLL/1("cos(wrt)*, sin(wrt)*") -> SPWM (Treg)2/7("cos(wrt)*, sin(wrt)*")
  Vs* [V]/1 -> SPWM (Treg)2/2(Vs* [V])
  SA,SB,SC,Se2/1(SA1pn) -> Mux1/1
  SA,SB,SC,Se2/2(SA2pn) -> Mux1/2
  SA,SB,SC,Se2/3(SB1pn) -> Mux1/3
  SA,SB,SC,Se2/4(SB2pn) -> Mux1/4
  SA,SB,SC,Se2/5(SC1pn) -> Mux1/5
  SA,SB,SC,Se2/6(SC2pn) -> Mux1/6
  SxA,SxB,SxC1/1("triangle (N) ") -> SA,SB,SC,Se2/2(triangle (N))
  Vdcpn [V]/1 -> input filter1/1(In1)
  vCf [V]/1 -> input filter1/2(In2)
  iLf [A]/1 -> input filter1/3(In3)
  iLoad [A]/1 -> input filter1/4(In4)
  3p PLL/2((wrt)* [deg]) -> Terminator/1
  input filter1/1(Out1) -> SPWM (Treg)2/3(Vdcpn [V])
  input filter1/2(Out2) -> SPWM (Treg)2/4(vCf [V])
  input filter1/3(Out3) -> SPWM (Treg)2/5(iLf [A])
  input filter1/4(Out4) -> SPWM (Treg)2/6(iLoad [A])
  SxA,SxB,SxC3/3(trigREG) -> SPWM (Treg)2/Trigger
  Data Type Conversion1/1 -> [VSIen], SPWM (Treg)2/1(En.)
  SPWM (Treg)2/1(vAM [pu]) -> Shadow Registers1/1(vAM |pu])
  SPWM (Treg)2/2(vBM [pu]) -> Shadow Registers1/2(vBM |pu])
  SPWM (Treg)2/3(vCM [pu]) -> Shadow Registers1/3(vCM |pu])
  SxA,SxB,SxC3/2(trigPWM_max/min) -> Shadow Registers1/Trigger
  Step/1 -> SPWM (Treg)2/8(startHC)
  Shadow Registers1/1(vAM [pu]) -> SA,SB,SC,Se2/3(vAM [pu])
  Shadow Registers1/2(vBM [pu]) -> SA,SB,SC,Se2/4(vBM [pu])
  Shadow Registers1/3(vCM [pu]) -> SA,SB,SC,Se2/5(vCM [pu])
  SxA,SxB,SxC3/1("triangle (P) ") -> SA,SB,SC,Se2/1(triangle (P))
  SPWM (Treg)2/4(vref [V]) -> vref/1
  SPWM (Treg)2/5(iref [A]) -> iref/1

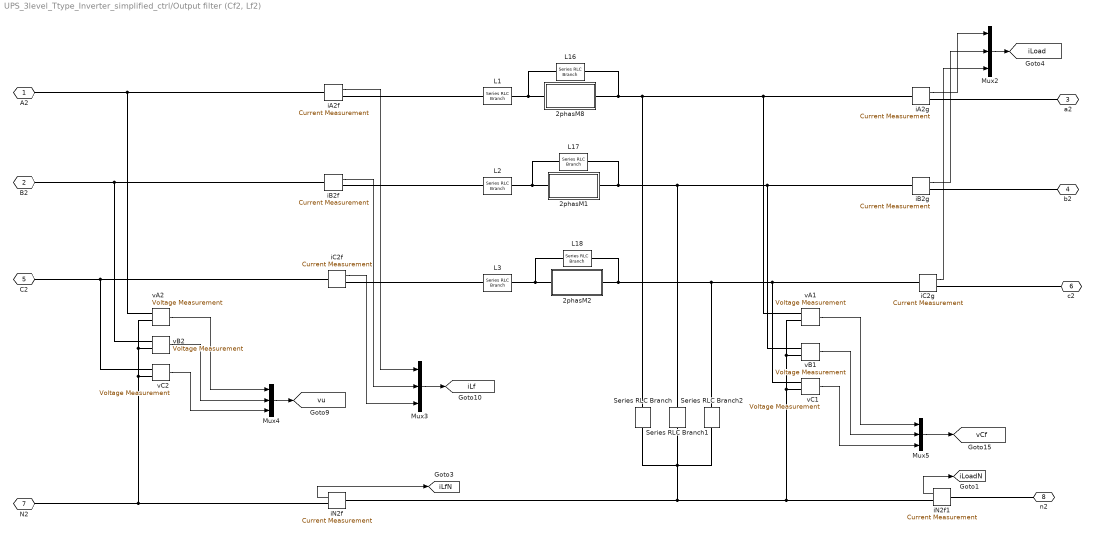
== system UPS_3level_Ttype_Inverter_simplified_ctrl/Output filter (Cf2, Lf2) ==
  2phasM1 : Subsystem
  2phasM2 : Subsystem
  2phasM8 : Subsystem
  L1 : powerlib/Elements/Series RLC Branch  LConnTagsString=__new0  RConnTagsString=__new0  BranchType=R  Resistance=VSI.Rf  Inductance=PR.Lf  SetiL0=off  InitialCurrent=0  Capacitance=1.0  Setx0=off  InitialVoltage=0  Measurements=None
  L16 : powerlib/Elements/Series RLC Branch  LConnTagsString=__new0  RConnTagsString=__new0  BranchType=R  Resistance=VSI.RfFe  Inductance=PR.Lf  SetiL0=off  InitialCurrent=0  Capacitance=1.0  Setx0=off  InitialVoltage=0  Measurements=None
  L17 : powerlib/Elements/Series RLC Branch  LConnTagsString=__new0  RConnTagsString=__new0  BranchType=R  Resistance=VSI.RfFe  Inductance=PR.Lf  SetiL0=off  InitialCurrent=0  Capacitance=1.0  Setx0=off  InitialVoltage=0  Measurements=None
  L18 : powerlib/Elements/Series RLC Branch  LConnTagsString=__new0  RConnTagsString=__new0  BranchType=R  Resistance=VSI.RfFe  Inductance=PR.Lf  SetiL0=off  InitialCurrent=0  Capacitance=1.0  Setx0=off  InitialVoltage=0  Measurements=None
  L2 : powerlib/Elements/Series RLC Branch  LConnTagsString=__new0  RConnTagsString=__new0  BranchType=R  Resistance=VSI.Rf  Inductance=PR.Lf  SetiL0=off  InitialCurrent=0  Capacitance=1.0  Setx0=off  InitialVoltage=0  Measurements=None
  L3 : powerlib/Elements/Series RLC Branch  LConnTagsString=__new0  RConnTagsString=__new0  BranchType=R  Resistance=VSI.Rf  Inductance=PR.Lf  SetiL0=off  InitialCurrent=0  Capacitance=1.0  Setx0=off  InitialVoltage=0  Measurements=None
  Mux{2..5} (4 alike) : Mux  Inputs=3
  Series RLC Branch : powerlib/Elements/Series RLC Branch  LConnTagsString=__new0  RConnTagsString=__new0  BranchType=RC  Resistance=VSI.Rcf  Inductance=1e-3  SetiL0=off  InitialCurrent=0  Capacitance=VSI.Cf  Setx0=on  InitialVoltage=VSI.Vcf0  Measurements=None
  Series RLC Branch1 : powerlib/Elements/Series RLC Branch  LConnTagsString=__new0  RConnTagsString=__new0  BranchType=RC  Resistance=VSI.Rcf  Inductance=1e-3  SetiL0=off  InitialCurrent=0  Capacitance=VSI.Cf  Setx0=on  InitialVoltage=VSI.Vcf0  Measurements=None
  Series RLC Branch2 : powerlib/Elements/Series RLC Branch  LConnTagsString=__new0  RConnTagsString=__new0  BranchType=RC  Resistance=VSI.Rcf  Inductance=1e-3  SetiL0=off  InitialCurrent=0  Capacitance=VSI.Cf  Setx0=on  InitialVoltage=VSI.Vcf0  Measurements=None
  iA2f : powerlib/Measurements/Current Measurement  PhasorSimulation=off  OutputType=Complex  PSBequivalent=0
  iA2g : powerlib/Measurements/Current Measurement  PhasorSimulation=off  OutputType=Complex  PSBequivalent=0
  iB2f : powerlib/Measurements/Current Measurement  PhasorSimulation=off  OutputType=Complex  PSBequivalent=0
  iB2g : powerlib/Measurements/Current Measurement  PhasorSimulation=off  OutputType=Complex  PSBequivalent=0
  iC2f : powerlib/Measurements/Current Measurement  PhasorSimulation=off  OutputType=Complex  PSBequivalent=0
  iC2g : powerlib/Measurements/Current Measurement  PhasorSimulation=off  OutputType=Complex  PSBequivalent=0
  iN2f : powerlib/Measurements/Current Measurement  PhasorSimulation=off  OutputType=Complex  PSBequivalent=0
  iN2f1 : powerlib/Measurements/Current Measurement  PhasorSimulation=off  OutputType=Complex  PSBequivalent=0
  vA1 : powerlib/Measurements/Voltage Measurement  PhasorSimulation=off  OutputType=Complex  PSBequivalent=0
  vA2 : powerlib/Measurements/Voltage Measurement  PhasorSimulation=off  OutputType=Complex  PSBequivalent=0
  vB1 : powerlib/Measurements/Voltage Measurement  PhasorSimulation=off  OutputType=Complex  PSBequivalent=0
  vB2 : powerlib/Measurements/Voltage Measurement  PhasorSimulation=off  OutputType=Complex  PSBequivalent=0
  vC1 : powerlib/Measurements/Voltage Measurement  PhasorSimulation=off  OutputType=Complex  PSBequivalent=0
  vC2 : powerlib/Measurements/Voltage Measurement  PhasorSimulation=off  OutputType=Complex  PSBequivalent=0
  A2 : PMIOPort  Port=1  Side=Left
  B2 : PMIOPort  Port=2  Side=Left
  a2 : PMIOPort  Port=3  Side=Right
  b2 : PMIOPort  Port=4  Side=Right
  C2 : PMIOPort  Port=5  Side=Left
  c2 : PMIOPort  Port=6  Side=Right
  N2 : PMIOPort  Port=7  Side=Left
  n2 : PMIOPort  Port=8  Side=Right
  tag scope: iLf=global, iLfN=global, iLoad=global, iLoadN=global, vCf=global, vu=global
  wires:
  vA2/1 -> Mux4/1
  vB2/1 -> Mux4/2
  vC2/1 -> Mux4/3
  Mux4/1 -> [vu]
  iA2f/1 -> Mux3/1
  iB2f/1 -> Mux3/2
  iC2f/1 -> Mux3/3
  iN2f/1 -> [iLfN]
  Mux3/1 -> [iLf]
  vA1/1 -> Mux5/1
  vB1/1 -> Mux5/2
  vC1/1 -> Mux5/3
  Mux5/1 -> [vCf]
  iA2g/1 -> Mux2/1
  iB2g/1 -> Mux2/2
  iC2g/1 -> Mux2/3
  Mux2/1 -> [iLoad]
  iN2f1/1 -> [iLoadN]
  connections:
  iA2f/LConn1 -- A2/RConn1 -- vA2/LConn1
  iB2f/LConn1 -- B2/RConn1 -- vB2/LConn1
  iC2f/LConn1 -- vC2/LConn1 -- C2/RConn1
  vB2/LConn2 -- vA2/LConn2 -- iN2f/RConn1 -- N2/RConn1 -- vC2/LConn2
  2phasM8/RConn1 -- iA2g/LConn1 -- vA1/LConn1 -- Series RLC Branch/LConn1 -- L16/RConn1
  2phasM1/RConn1 -- iB2g/LConn1 -- vB1/LConn1 -- Series RLC Branch1/LConn1 -- L17/RConn1
  2phasM2/RConn1 -- Series RLC Branch2/LConn1 -- iC2g/LConn1 -- vC1/LConn1 -- L18/RConn1
  iN2f/LConn1 -- iN2f1/RConn1 -- vC1/LConn2 -- vB1/LConn2 -- vA1/LConn2 -- Series RLC Branch1/RConn1 -- Series RLC Branch/RConn1 -- Series RLC Branch2/RConn1
  2phasM1/LConn1 -- L2/RConn1 -- L17/LConn1
  L2/LConn1 -- iB2f/RConn1
  L1/RConn1 -- 2phasM8/LConn1 -- L16/LConn1
  L1/LConn1 -- iA2f/RConn1
  2phasM2/LConn1 -- L3/RConn1 -- L18/LConn1
  L3/LConn1 -- iC2f/RConn1
  iC2g/RConn1 -- c2/RConn1
  iA2g/RConn1 -- a2/RConn1
  iB2g/RConn1 -- b2/RConn1
  iN2f1/LConn1 -- n2/RConn1

== system UPS_3level_Ttype_Inverter_simplified_ctrl/Subsystem6 ==
  2 [s]1 : Constant  Value=VSI.t0 + 0.05
  Ideal Switch : powerlib/Power Electronics/Ideal Switch  Ron=0.001  Lon=0  IC=0  Rs=1e6  Cs=inf  Measurements=off
  Relational Operator1 : RelationalOperator  OutDataTypeStr=boolean
  in : PMIOPort  Port=1  Side=Left
  out : PMIOPort  Port=2  Side=Right
  wires:
  [tT] -> Relational Operator1/1
  2 [s]1/1 -> Relational Operator1/2
  Relational Operator1/1 -> Ideal Switch/1
  connections:
  Ideal Switch/LConn1 -- in/RConn1
  Ideal Switch/RConn1 -- out/RConn1

== system UPS_3level_Ttype_Inverter_simplified_ctrl/Subsystem7 ==
  2 [s]1 : Constant  Value=VSI.t0 + 0.05
  Ideal Switch : powerlib/Power Electronics/Ideal Switch  Ron=0.001  Lon=0  IC=0  Rs=1e6  Cs=inf  Measurements=off
  Relational Operator1 : RelationalOperator  OutDataTypeStr=boolean
  in : PMIOPort  Port=1  Side=Left
  out : PMIOPort  Port=2  Side=Right
  wires:
  [tT] -> Relational Operator1/1
  2 [s]1/1 -> Relational Operator1/2
  Relational Operator1/1 -> Ideal Switch/1
  connections:
  Ideal Switch/LConn1 -- in/RConn1
  Ideal Switch/RConn1 -- out/RConn1

== system UPS_3level_Ttype_Inverter_simplified_ctrl/Subsystem8 ==
  2 [s]1 : Constant  Value=VSI.t0 + 0.05
  Ideal Switch : powerlib/Power Electronics/Ideal Switch  Ron=0.001  Lon=0  IC=0  Rs=1e6  Cs=inf  Measurements=off
  Relational Operator1 : RelationalOperator  OutDataTypeStr=boolean
  in : PMIOPort  Port=1  Side=Left
  out : PMIOPort  Port=2  Side=Right
  wires:
  [tT] -> Relational Operator1/1
  2 [s]1/1 -> Relational Operator1/2
  Relational Operator1/1 -> Ideal Switch/1
  connections:
  Ideal Switch/LConn1 -- in/RConn1
  Ideal Switch/RConn1 -- out/RConn1

== system UPS_3level_Ttype_Inverter_simplified_ctrl/4-leg PWM1/Subsystem3 ==
  2 [s]1 : Constant  Value=VSI.t0 + 0.05
  Ideal Switch : powerlib/Power Electronics/Ideal Switch  Ron=0.001  Lon=0  IC=0  Rs=1e6  Cs=inf  Measurements=off
  Relational Operator1 : RelationalOperator  OutDataTypeStr=boolean
  in : PMIOPort  Port=1  Side=Left
  out : PMIOPort  Port=2  Side=Right
  wires:
  [tT] -> Relational Operator1/1
  2 [s]1/1 -> Relational Operator1/2
  Relational Operator1/1 -> Ideal Switch/1
  connections:
  Ideal Switch/RConn1 -- out/RConn1
  Ideal Switch/LConn1 -- in/RConn1

== system UPS_3level_Ttype_Inverter_simplified_ctrl/4-leg PWM2/Subsystem1 ==
  2 [s]1 : Constant  Value=VSI.t0 + 0.05
  Ideal Switch : powerlib/Power Electronics/Ideal Switch  Ron=0.001  Lon=0  IC=0  Rs=1e6  Cs=inf  Measurements=off
  Relational Operator1 : RelationalOperator  OutDataTypeStr=boolean
  in : PMIOPort  Port=1  Side=Left
  out : PMIOPort  Port=2  Side=Right
  wires:
  Relational Operator1/1 -> Ideal Switch/1
  2 [s]1/1 -> Relational Operator1/2
  [tT] -> Relational Operator1/1
  connections:
  Ideal Switch/LConn1 -- in/RConn1
  Ideal Switch/RConn1 -- out/RConn1

== system UPS_3level_Ttype_Inverter_simplified_ctrl/4-leg PWM2/Subsystem2 ==
  2 [s]1 : Constant  Value=VSI.t0 + 0.05
  Ideal Switch : powerlib/Power Electronics/Ideal Switch  Ron=0.001  Lon=0  IC=0  Rs=1e6  Cs=inf  Measurements=off
  Relational Operator1 : RelationalOperator  OutDataTypeStr=boolean
  in : PMIOPort  Port=1  Side=Left
  out : PMIOPort  Port=2  Side=Right
  wires:
  [tT] -> Relational Operator1/1
  2 [s]1/1 -> Relational Operator1/2
  Relational Operator1/1 -> Ideal Switch/1
  connections:
  Ideal Switch/RConn1 -- out/RConn1
  Ideal Switch/LConn1 -- in/RConn1

== system UPS_3level_Ttype_Inverter_simplified_ctrl/4-leg PWM2/Subsystem3 ==
  2 [s]1 : Constant  Value=VSI.t0 + 0.05
  Ideal Switch : powerlib/Power Electronics/Ideal Switch  Ron=0.001  Lon=0  IC=0  Rs=1e6  Cs=inf  Measurements=off
  Relational Operator1 : RelationalOperator  OutDataTypeStr=boolean
  in : PMIOPort  Port=1  Side=Left
  out : PMIOPort  Port=2  Side=Right
  wires:
  [tT] -> Relational Operator1/1
  2 [s]1/1 -> Relational Operator1/2
  Relational Operator1/1 -> Ideal Switch/1
  connections:
  Ideal Switch/RConn1 -- out/RConn1
  Ideal Switch/LConn1 -- in/RConn1

== system UPS_3level_Ttype_Inverter_simplified_ctrl/Output Switch/Subsystem4 ==
  on/off : Inport
  Ideal Switch : powerlib/Power Electronics/Ideal Switch  Ron=0.0001  Lon=0  IC=0  Rs=1e6  Cs=inf  Measurements=off
  in : PMIOPort  Port=1  Side=Left
  out : PMIOPort  Port=2  Side=Right
  wires:
  on/off/1 -> Ideal Switch/1
  connections:
  out/RConn1 -- Ideal Switch/RConn1
  in/RConn1 -- Ideal Switch/LConn1

== system UPS_3level_Ttype_Inverter_simplified_ctrl/Output Switch/Subsystem5 ==
  on/off : Inport
  Ideal Switch : powerlib/Power Electronics/Ideal Switch  Ron=0.0001  Lon=0  IC=0  Rs=1e6  Cs=inf  Measurements=off
  in : PMIOPort  Port=1  Side=Left
  out : PMIOPort  Port=2  Side=Right
  wires:
  on/off/1 -> Ideal Switch/1
  connections:
  out/RConn1 -- Ideal Switch/RConn1
  in/RConn1 -- Ideal Switch/LConn1

== system UPS_3level_Ttype_Inverter_simplified_ctrl/Output Switch/Subsystem7 ==
  on/off : Inport
  Ideal Switch : powerlib/Power Electronics/Ideal Switch  Ron=0.0001  Lon=0  IC=0  Rs=1e6  Cs=inf  Measurements=off
  in : PMIOPort  Port=1  Side=Left
  out : PMIOPort  Port=2  Side=Right
  wires:
  on/off/1 -> Ideal Switch/1
  connections:
  out/RConn1 -- Ideal Switch/RConn1
  in/RConn1 -- Ideal Switch/LConn1

== system UPS_3level_Ttype_Inverter_simplified_ctrl/Output Inverter Control System SRF(dq0) - SPWM /3p PLL ==
  2 [s]1 : Constant
  2 [s]2 : Constant  Value=S.fi0h1
  2 [s]3 : Constant  Value=2*pi
  Add5 : Sum
  Gain : Gain  Gain=180/pi
  Math Function : Math  Operator=mod  SaturateOnIntegerOverflow=on
  Mux4 : Mux  Inputs=2
  "va, vb" : Subsystem
  "cos(wrt)*, sin(wrt)*" : Outport
  (wrt)* [deg] : Outport  Port=2
  wires:
  Gain/1 -> "va, vb"/2("wrt* [deg] "), (wrt)* [deg]/1
  2 [s]1/1 -> "va, vb"/1(Vm* [pu])
  "va, vb"/1(cos(wrt)*) -> Mux4/1
  "va, vb"/2(sin(wrt)*) -> Mux4/2
  Mux4/1 -> "cos(wrt)*, sin(wrt)*"/1
  Add5/1 -> Math Function/1
  2 [s]2/1 -> Add5/2
  Math Function/1 -> Gain/1
  [wrtREFT] -> Add5/1
  2 [s]3/1 -> Math Function/2

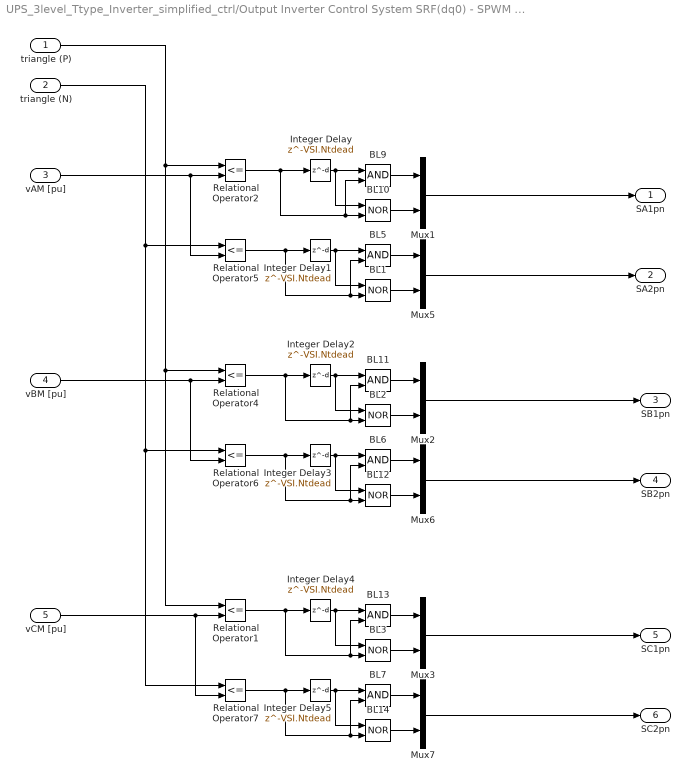
== system UPS_3level_Ttype_Inverter_simplified_ctrl/Output Inverter Control System SRF(dq0) - SPWM /SA,SB,SC,Se2 ==
  triangle (P) : Inport
  triangle (N) : Inport  Port=2
  vAM [pu] : Inport  Port=3
  vBM [pu] : Inport  Port=4
  vCM [pu] : Inport  Port=5
  BL{1..3,10,12,14} (6 alike) : Logic  Operator=NOR
  BL{5..7,9,11,13} (6 alike) : Logic
  Integer Delay{,1..5} (6 alike) : Delay  DelayLength=VSI.Ntdead  InitialCondition=0  InputProcessing=Inherited
  Mux{1..3,5..7} (6 alike) : Mux  Inputs=2
  Relational Operator{1..2,4..7} (6 alike) : RelationalOperator  Operator=<=  InputSameDT=on
  SA1pn : Outport
  SA2pn : Outport  Port=2
  SB1pn : Outport  Port=3
  SB2pn : Outport  Port=4
  SC1pn : Outport  Port=5
  SC2pn : Outport  Port=6
  wires:
  triangle (P)/1 -> Relational Operator2/1, Relational Operator4/1, Relational Operator1/1
  vAM [pu]/1 -> Relational Operator2/2, Relational Operator5/2
  vBM [pu]/1 -> Relational Operator4/2, Relational Operator6/2
  Mux1/1 -> SA1pn/1
  triangle (N)/1 -> Relational Operator5/1, Relational Operator6/1, Relational Operator7/1
  vCM [pu]/1 -> Relational Operator1/2, Relational Operator7/2
  Integer Delay/1 -> BL9/1, BL10/1
  BL9/1 -> Mux1/1
  BL10/1 -> Mux1/2
  Relational Operator2/1 -> Integer Delay/1, BL10/2, BL9/2
  Integer Delay1/1 -> BL5/1, BL1/1
  BL5/1 -> Mux5/1
  BL1/1 -> Mux5/2
  Relational Operator5/1 -> Integer Delay1/1, BL1/2, BL5/2
  Mux5/1 -> SA2pn/1
  Integer Delay2/1 -> BL11/1, BL2/1
  BL11/1 -> Mux2/1
  BL2/1 -> Mux2/2
  Relational Operator4/1 -> Integer Delay2/1, BL2/2, BL11/2
  Mux2/1 -> SB1pn/1
  Integer Delay3/1 -> BL6/1, BL12/1
  BL6/1 -> Mux6/1
  BL12/1 -> Mux6/2
  Relational Operator6/1 -> Integer Delay3/1, BL12/2, BL6/2
  Mux6/1 -> SB2pn/1
  Integer Delay4/1 -> BL13/1, BL3/1
  BL13/1 -> Mux3/1
  BL3/1 -> Mux3/2
  Relational Operator1/1 -> Integer Delay4/1, BL3/2, BL13/2
  Mux3/1 -> SC1pn/1
  Integer Delay5/1 -> BL7/1, BL14/1
  BL7/1 -> Mux7/1
  BL14/1 -> Mux7/2
  Relational Operator7/1 -> Integer Delay5/1, BL14/2, BL7/2
  Mux7/1 -> SC2pn/1

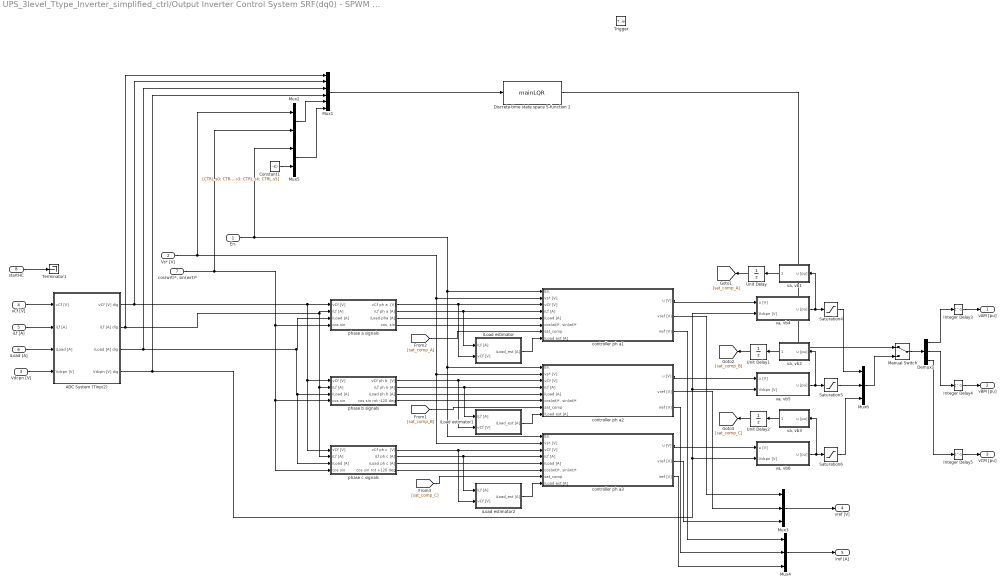
== system UPS_3level_Ttype_Inverter_simplified_ctrl/Output Inverter Control System SRF(dq0) - SPWM /SPWM (Treg)2 ==
  En. : Inport
  Vs* [V] : Inport  Port=2
  Vdcpn [V] : Inport  Port=3
  vCf [V] : Inport  Port=4
  iLf [A] : Inport  Port=5
  iLoad [A] : Inport  Port=6
  "cos(wrt)*, sin(wrt)*" : Inport  Port=7
  startHC : Inport  Port=8
  Trigger : TriggerPort
  " ADC System (Tinp/2)" : Subsystem
  Constant1 : Constant  Value=[CTRL.s0; CTRL.s1; CTRL.s2; CTRL.s3; CTRL.s4; CTRL.s5]
  Demux1 : Demux  Outputs=3
  Discrete-time state space S-function 2 : S-Function  FunctionName=mainLQR  EnableBusSupport=off  mask(S-function: dsfunc){}
      mask help: This is a S-function which does the discrete state space system.
      mask Display: disp('x(n+1) = Ax(n) + Bu(n)\n y(n)     = Cx(n) + Du(n) ');
  Integer Delay3 : Delay  DelayLength=1  InitialCondition=0  InputProcessing=Inherited
  Integer Delay4 : Delay  DelayLength=1  InitialCondition=0  InputProcessing=Inherited
  Integer Delay5 : Delay  DelayLength=1  InitialCondition=0  InputProcessing=Inherited
  Manual Switch : ManualSwitch
  Mux1 : Mux  Inputs=6
  Mux2 : Mux  Inputs=2
  Mux3 : Mux  Inputs=3
  Mux4 : Mux  Inputs=3
  Mux5 : Mux  Inputs=2
  Mux6 : Mux  Inputs=3
  Saturation4 : Saturate  UpperLimit=1  LowerLimit=-1
  Saturation5 : Saturate  UpperLimit=1  LowerLimit=-1
  Saturation6 : Saturate  UpperLimit=1  LowerLimit=-1
  Terminator1 : Terminator
  Unit Delay : UnitDelay  SampleTime=-1
  Unit Delay1 : UnitDelay  SampleTime=-1
  Unit Delay2 : UnitDelay  SampleTime=-1
  controller ph a1 : Subsystem
  controller ph a2 : Subsystem
  controller ph a3 : Subsystem
  iLoad estimator : Subsystem
  iLoad estimator1 : Subsystem
  iLoad estimator2 : Subsystem
  phase a signals : Subsystem
  phase b signals : Subsystem
  phase c signals : Subsystem
  "va, vb1" : Subsystem
  "va, vb2" : Subsystem
  "va, vb3" : Subsystem
  "va, vb4" : Subsystem
  "va, vb5" : Subsystem
  "va, vb6" : Subsystem
  vAM [pu] : Outport
  vBM [pu] : Outport  Port=2
  vCM [pu] : Outport  Port=3
  vref [V] : Outport  Port=4
  iref [A] : Outport  Port=5
  wires:
  Vdcpn [V]/1 -> " ADC System (Tinp/2)"/4(Vdcpn [V])
  vCf [V]/1 -> " ADC System (Tinp/2)"/1(vCf [V])
  iLf [A]/1 -> " ADC System (Tinp/2)"/2(iLf [A])
  iLoad [A]/1 -> " ADC System (Tinp/2)"/3(iLoad [A])
  En./1 -> controller ph a1/1(En.), controller ph a3/1(En.), controller ph a2/1(En.), Mux5/1
  startHC/1 -> Terminator1/1
  "va, vb4"/1(u [pu]) -> "va, vb1"/1(u [pu]), Saturation4/1
  Saturation4/1 -> Mux6/1
  " ADC System (Tinp/2)"/1(vCf [V] dig) -> Mux1/2, phase c signals/1(vCf [V]), phase b signals/1(vCf [V]), phase a signals/1(vCf [V])
  Saturation5/1 -> Mux6/2
  controller ph a2/1(u [V]) -> "va, vb5"/1(u [V])
  Saturation6/1 -> Mux6/3
  controller ph a3/1(u [V]) -> "va, vb6"/1(u [V])
  phase b signals/3(iLoad ph b [A]) -> controller ph a2/5(iLoad [A])
  phase c signals/3(iLoad ph c [A]) -> controller ph a3/5(iLoad [A])
  Integer Delay3/1 -> vAM [pu]/1
  Integer Delay4/1 -> vBM [pu]/1
  Integer Delay5/1 -> vCM [pu]/1
  phase b signals/1(vCf ph b  [V]) -> controller ph a2/3(vCf [V]), iLoad estimator1/2(vCf [V])
  phase b signals/2(iLf ph b [A]) -> iLoad estimator1/1(iLf [A]), controller ph a2/4(iLf [A])
  phase c signals/1(vCf ph c  [V]) -> iLoad estimator2/2(vCf [V]), controller ph a3/3(vCf [V])
  phase c signals/2(iLf ph c [A]) -> iLoad estimator2/1(iLf [A]), controller ph a3/4(iLf [A])
  phase a signals/3(iLoad pha [A]) -> controller ph a1/5(iLoad [A])
  phase a signals/2(iLf ph a [A]) -> iLoad estimator/1(iLf [A]), controller ph a1/4(iLf [A])
  phase a signals/1(vCf ph a  [V]) -> controller ph a1/3(vCf [V]), iLoad estimator/2(vCf [V])
  phase a signals/4("cos, sin") -> controller ph a1/6("cos(wt)*, sin(wt)*")
  phase b signals/4(cos sin rot -120 deg) -> controller ph a2/6("cos(wt)*, sin(wt)*")
  phase c signals/4(cos sin rot +120 deg) -> controller ph a3/6("cos(wt)*, sin(wt)*")
  " ADC System (Tinp/2)"/3(iLoad [A] dig) -> phase c signals/3(iLoad [A]), phase b signals/3(iLoad [A]), phase a signals/3(iLoad [A]), Mux1/3
  controller ph a1/1(u [V]) -> "va, vb4"/1(u [V])
  controller ph a1/2(vref [V]) -> Mux3/1
  "va, vb1"/1(sat_comp) -> Unit Delay/1
  Unit Delay/1 -> [sat_comp_A]
  "va, vb2"/1(sat_comp) -> Unit Delay1/1
  Unit Delay1/1 -> [sat_comp_B]
  "va, vb3"/1(sat_comp) -> Unit Delay2/1
  Unit Delay2/1 -> [sat_comp_C]
  "va, vb5"/1(u [pu]) -> "va, vb2"/1(u [pu]), Saturation5/1
  "va, vb6"/1(u [pu]) -> "va, vb3"/1(u [pu]), Saturation6/1
  [sat_comp_A] -> controller ph a1/7(sat_comp)
  [sat_comp_B] -> controller ph a2/7(sat_comp)
  [sat_comp_C] -> controller ph a3/7(sat_comp)
  Constant1/1 -> Mux5/2
  "cos(wrt)*, sin(wrt)*"/1 -> Mux2/2, phase c signals/4(cos sin), phase b signals/4(cos sin), phase a signals/4(cos sin)
  Mux2/1 -> Mux1/5
  Mux5/1 -> Mux1/6
  " ADC System (Tinp/2)"/2(iLf [A] dig) -> Mux1/1, phase c signals/2(iLf [A]), phase b signals/2(iLf [A]), phase a signals/2(iLf [A])
  " ADC System (Tinp/2)"/4(Vdcpn [V] dig) -> Mux1/4, "va, vb4"/2(Vdcpn [V]), "va, vb5"/2(Vdcpn [V]), "va, vb6"/2(Vdcpn [V])
  Vs* [V]/1 -> Mux2/1, controller ph a1/2(vs* [V]), controller ph a3/2(vs* [V]), controller ph a2/2(vs* [V])
  Mux1/1 -> Discrete-time state space S-function 2/1
  Discrete-time state space S-function 2/1 -> Manual Switch/1
  Manual Switch/1 -> Demux1/1
  Mux6/1 -> Manual Switch/2
  Demux1/1 -> Integer Delay3/1
  Demux1/2 -> Integer Delay4/1
  Demux1/3 -> Integer Delay5/1
  iLoad estimator/1(iLoad_est [A]) -> controller ph a1/8(iLoad est [A])
  iLoad estimator1/1(iLoad_est [A]) -> controller ph a2/8(iLoad est [A])
  iLoad estimator2/1(iLoad_est [A]) -> controller ph a3/8(iLoad est [A])
  Mux3/1 -> vref [V]/1
  controller ph a2/2(vref [V]) -> Mux3/2
  controller ph a3/2(vref [V]) -> Mux3/3
  Mux4/1 -> iref [A]/1
  controller ph a3/3(iref [V]) -> Mux4/3
  controller ph a2/3(iref [V]) -> Mux4/2
  controller ph a1/3(iref [V]) -> Mux4/1

== system UPS_3level_Ttype_Inverter_simplified_ctrl/Output Inverter Control System SRF(dq0) - SPWM /Shadow Registers1 ==
  vAM |pu] : Inport
  vBM |pu] : Inport  Port=2
  vCM |pu] : Inport  Port=3
  Trigger : TriggerPort
  vAM [pu] : Outport
  vBM [pu] : Outport  Port=2
  vCM [pu] : Outport  Port=3
  wires:
  vCM |pu]/1 -> vCM [pu]/1
  vBM |pu]/1 -> vBM [pu]/1
  vAM |pu]/1 -> vAM [pu]/1

== system UPS_3level_Ttype_Inverter_simplified_ctrl/Output Inverter Control System SRF(dq0) - SPWM /SxA,SxB,SxC1 ==
  triangle : simulink/Sources/Repeating Sequence  rep_seq_t="[0  VSI.Tinp/2  VSI.Tinp]"  rep_seq_y="[0   -1   0]"
  "triangle (N) " : Outport
  wires:
  triangle/1 -> "triangle (N) "/1

== system UPS_3level_Ttype_Inverter_simplified_ctrl/Output Inverter Control System SRF(dq0) - SPWM /SxA,SxB,SxC3 ==
  Constant7 : Constant  Value=0.99
  Constant8 : Constant  Value=0.01
  Data Type Conversion1 : DataTypeConversion  OutDataTypeStr=boolean  SaturateOnIntegerOverflow=on  RndMeth=Zero
  Data Type Conversion2 : DataTypeConversion  OutDataTypeStr=boolean  SaturateOnIntegerOverflow=on  RndMeth=Zero
  Logical Operator : Logic  Operator=OR  AllPortsSameDT=off  OutDataTypeStr=boolean
  Pulse Generaor : DiscretePulseGenerator  PulseType=Time based  TimeSource=Use external signal  Period=VSI.Treg  PulseWidth=50
  Pulse Generaor1 : DiscretePulseGenerator  PulseType=Time based  TimeSource=Use external signal  Period=VSI.Tinp/2  PulseWidth=50
  Relational Operator1 : RelationalOperator  Operator=<=  InputSameDT=on
  Relational Operator2 : RelationalOperator  InputSameDT=on
  triangle : simulink/Sources/Repeating Sequence  rep_seq_t="[0  VSI.Tinp/2  VSI.Tinp]"  rep_seq_y="[1   0   1]"
  "triangle (P) " : Outport
  trigPWM_max/min : Outport  Port=2
  trigREG : Outport  Port=3
  wires:
  triangle/1 -> "triangle (P) "/1, Relational Operator1/1, Relational Operator2/1
  Constant7/1 -> Relational Operator2/2
  Constant8/1 -> Relational Operator1/2
  Pulse Generaor/1 -> Data Type Conversion2/1
  [tT] -> Pulse Generaor/1
  Data Type Conversion2/1 -> trigREG/1
  Relational Operator1/1 -> Logical Operator/1
  Relational Operator2/1 -> Logical Operator/2
  Logical Operator/1 -> ?
  Pulse Generaor1/1 -> Data Type Conversion1/1
  [tT] -> Pulse Generaor1/1
  Data Type Conversion1/1 -> trigPWM_max/min/1
